simulink model "airspeed_controller"  (R2018b)
settings: Solver=FixedStepAuto  StartTime=0.0  StopTime=200  FixedStep=0.001  RelTol=1e-3
model workspace (MAT data in the model file):
  Cd = 0.18
  climb_max = 5
  g_common = 9.81
  mass_plane = 1.5
  nomThr = 0
  rou = 1.225
  sink_max = 1
  timeConstThrot = 8
libraries: simulink x2
settings Model: Creator=lee  LastModifiedBy=lee

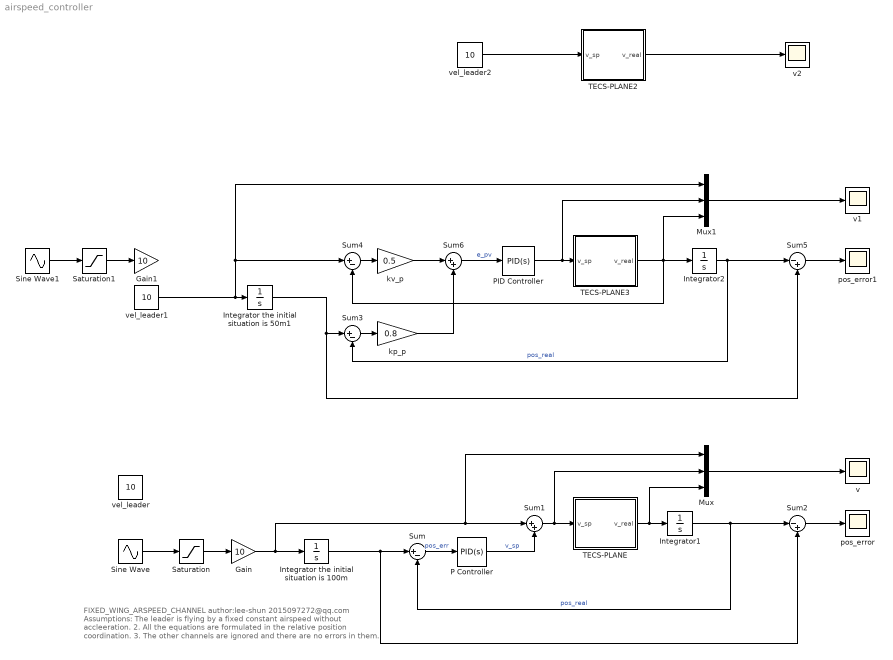
== system airspeed_controller ==
  note: FIXED_WING_ARSPEED_CHANNEL
      |
      | author:lee-shun 2015097272@qq.com
      |
      | Assumptions:
      |
      | The leader is flying by a fixed constant airspeed without accleeration.
      | 2. All the equations are formulated in the relative position coordination.
      | 3. The other channels are ignored and there are no errors in them.
  Gain : Gain  Gain=10
  Gain1 : Gain  Gain=10
  Integrator the initial situation is 100m : Integrator  InitialCondition=50  IgnoreLimit=on
  Integrator the initial situation is 50m1 : Integrator  InitialCondition=50  IgnoreLimit=on
  Integrator1 : Integrator
  Integrator2 : Integrator
  Mux : Mux  Inputs=3
  Mux1 : Mux  Inputs=3
  P Controller : simulink/Continuous/PID Controller  Controller=PID  Form=Parallel  TimeDomain=Continuous-time  SampleTime=-1  IntegratorMethod=Forward Euler  FilterMethod=Forward Euler  ControllerParametersSource=internal  P=0.02  I=0  D=0.0  UseFilter=on  N=100  TunerSelectOption=Transfer Function Based (PID Tuner App)  InitialConditionSource=internal  InitialConditionForIntegrator=0  InitialConditionForFilter=0  DifferentiatorICPrevScaledInput=0  ExternalReset=none  TrackingMode=off  Kt=1  LimitOutput=off  UpperSaturationLimit=inf  LowerSaturationLimit=-inf  LinearizeAsGain=on  AntiWindupMode=none  Kb=1  POutMin=[]  POutMax=[]  IOutMin=[]  IOutMax=[]  DOutMin=[]  DOutMax=[]  NOutMin=[]  NOutMax=[]  SumOutMin=[]  SumOutMax=[]  SaturationOutMin=[]  SaturationOutMax=[]  PParamMin=[]  PParamMax=[]  IParamMin=[]  IParamMax=[]  DParamMin=[]  DParamMax=[]  NParamMin=[]  NParamMax=[]  KbParamMin=[]  KbParamMax=[]  KtParamMin=[]  KtParamMax=[]  KbOutMin=[]  KbOutMax=[]  KtOutMin=[]  KtOutMax=[]  IntegratorOutMin=[]  IntegratorOutMax=[]  FilterOutMin=[]  FilterOutMax=[]  SumI1OutMin=[]  SumI1OutMax=[]  SumI2OutMin=[]  SumI2OutMax=[]  SumI3OutMin=[]  SumI3OutMax=[]  SumI4OutMin=[]  SumI4OutMax=[]  SumDOutMin=[]  SumDOutMax=[]  DifferentiatorOutMin=[]  DifferentiatorOutMax=[]  FilterDiffOutCoefMin=[]  FilterDiffOutCoefMax=[]  ReciprocalOutMin=[]  ReciprocalOutMax=[]  SumDenOutMin=[]  SumDenOutMax=[]  SumNumOutMin=[]  SumNumOutMax=[]  DivideOutMin=[]  DivideOutMax=[]  IntegratorContinuousStateAttributes=''  IntegratorStateMustResolveToSignalObject=off  IntegratorRTWStateStorageClass=Auto  FilterContinuousStateAttributes=''  FilterStateMustResolveToSignalObject=off  FilterRTWStateStorageClass=Auto  ParallelPVariant=InternalParameters  IdealPVariant=Disabled  IVariant=InternalParameters  DVariant=InternalParameters  IntegratorVariant=Continuous  SatVariant=Disabled  AWVariant=Passthrough  PCopyVariant=Disabled  TRVariant=Disabled  FdbkBlocksVariant=Forward  IdealPFdbkVariant=Disabled  SatFdbkVariant=Disabled  DerivativeFilterVariant=ContFilter  NVariant=InternalParameters  NCopyVariant=Disabled  FilterICVariant=InternalICsFilter  IntegratorICVariant=InternalICs  ExternalResetVariant=Disabled  TRSumVariant=Passthrough  SumFdbkVariant=Disabled  SumVariant=Sum_PID
  PID Controller : simulink/Continuous/PID Controller  Controller=PID  Form=Parallel  TimeDomain=Continuous-time  SampleTime=-1  IntegratorMethod=Forward Euler  FilterMethod=Forward Euler  ControllerParametersSource=internal  P=0.3  I=0.01  D=0  UseFilter=on  N=100  TunerSelectOption=Transfer Function Based (PID Tuner App)  InitialConditionSource=internal  InitialConditionForIntegrator=0  InitialConditionForFilter=0  DifferentiatorICPrevScaledInput=0  ExternalReset=none  TrackingMode=off  Kt=1  LimitOutput=off  UpperSaturationLimit=inf  LowerSaturationLimit=-inf  LinearizeAsGain=on  AntiWindupMode=none  Kb=1  POutMin=[]  POutMax=[]  IOutMin=[]  IOutMax=[]  DOutMin=[]  DOutMax=[]  NOutMin=[]  NOutMax=[]  SumOutMin=[]  SumOutMax=[]  SaturationOutMin=[]  SaturationOutMax=[]  PParamMin=[]  PParamMax=[]  IParamMin=[]  IParamMax=[]  DParamMin=[]  DParamMax=[]  NParamMin=[]  NParamMax=[]  KbParamMin=[]  KbParamMax=[]  KtParamMin=[]  KtParamMax=[]  KbOutMin=[]  KbOutMax=[]  KtOutMin=[]  KtOutMax=[]  IntegratorOutMin=[]  IntegratorOutMax=[]  FilterOutMin=[]  FilterOutMax=[]  SumI1OutMin=[]  SumI1OutMax=[]  SumI2OutMin=[]  SumI2OutMax=[]  SumI3OutMin=[]  SumI3OutMax=[]  SumI4OutMin=[]  SumI4OutMax=[]  SumDOutMin=[]  SumDOutMax=[]  DifferentiatorOutMin=[]  DifferentiatorOutMax=[]  FilterDiffOutCoefMin=[]  FilterDiffOutCoefMax=[]  ReciprocalOutMin=[]  ReciprocalOutMax=[]  SumDenOutMin=[]  SumDenOutMax=[]  SumNumOutMin=[]  SumNumOutMax=[]  DivideOutMin=[]  DivideOutMax=[]  IntegratorContinuousStateAttributes=''  IntegratorStateMustResolveToSignalObject=off  IntegratorRTWStateStorageClass=Auto  FilterContinuousStateAttributes=''  FilterStateMustResolveToSignalObject=off  FilterRTWStateStorageClass=Auto  ParallelPVariant=InternalParameters  IdealPVariant=Disabled  IVariant=InternalParameters  DVariant=InternalParameters  IntegratorVariant=Continuous  SatVariant=Disabled  AWVariant=Passthrough  PCopyVariant=Disabled  TRVariant=Disabled  FdbkBlocksVariant=Forward  IdealPFdbkVariant=Disabled  SatFdbkVariant=Disabled  DerivativeFilterVariant=ContFilter  NVariant=InternalParameters  NCopyVariant=Disabled  FilterICVariant=InternalICsFilter  IntegratorICVariant=InternalICs  ExternalResetVariant=Disabled  TRSumVariant=Passthrough  SumFdbkVariant=Disabled  SumVariant=Sum_PID
  Saturation : Saturate  UpperLimit=1  LowerLimit=0.2
  Saturation1 : Saturate  UpperLimit=1  LowerLimit=0.2
  Sine Wave : Sin  Frequency=0.1  SampleTime=0
  Sine Wave1 : Sin  Frequency=0.1  SampleTime=0
  Sum : Sum  Inputs=|+-
  Sum1 : Sum  Inputs=|++
  Sum2 : Sum  Inputs=|-+
  Sum3 : Sum  Inputs=|+-
  Sum4 : Sum  Inputs=|+-
  Sum5 : Sum  Inputs=|-+
  Sum6 : Sum  Inputs=|++
  TECS-PLANE : Subsystem
  TECS-PLANE2 : Subsystem
  TECS-PLANE3 : Subsystem
  kp_p : Gain  Gain=0.8
  kv_p : Gain  Gain=0.5
  pos_error : Scope
  pos_error1 : Scope
  v : Scope
  v1 : Scope
  v2 : Scope
  vel_leader : Constant  Value=10
  vel_leader1 : Constant  Value=10
  vel_leader2 : Constant  Value=10
  wires:
  Sum/1 -> P Controller/1  "pos_err"
  Integrator1/1 -> Sum/2, Sum2/1  "pos_real"
  Integrator the initial situation is 100m/1 -> Sum/1, Sum2/2
  TECS-PLANE/1(v_real) -> Mux/3, Integrator1/1
  P Controller/1 -> Sum1/2  "v_sp"
  Sum1/1 -> Mux/2, TECS-PLANE/1(v_sp)
  Sum2/1 -> pos_error/1
  Sine Wave/1 -> Saturation/1
  Saturation/1 -> Gain/1
  Gain/1 -> Mux/1, Sum1/1, Integrator the initial situation is 100m/1
  Mux/1 -> v/1
  Sum5/1 -> pos_error1/1
  Saturation1/1 -> Gain1/1
  Sine Wave1/1 -> Saturation1/1
  TECS-PLANE3/1(v_real) -> Integrator2/1, Mux1/3, Sum4/2
  Integrator2/1 -> Sum5/1, Sum3/2  "pos_real"
  Mux1/1 -> v1/1
  Integrator the initial situation is 50m1/1 -> Sum3/1, Sum5/2
  kv_p/1 -> Sum6/1
  Sum4/1 -> kv_p/1
  Sum3/1 -> kp_p/1
  kp_p/1 -> Sum6/2
  Sum6/1 -> PID Controller/1  "e_pv"
  PID Controller/1 -> TECS-PLANE3/1(v_sp), Mux1/2
  vel_leader1/1 -> Sum4/1, Mux1/1, Integrator the initial situation is 50m1/1
  vel_leader2/1 -> TECS-PLANE2/1(v_sp)
  TECS-PLANE2/1(v_real) -> v2/1

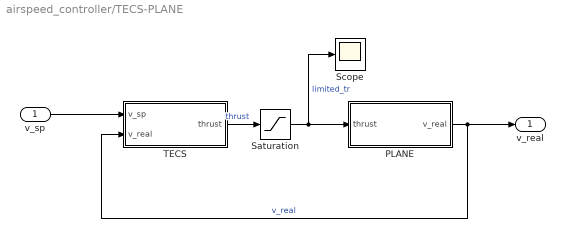
== system airspeed_controller/TECS-PLANE ==
  v_sp : Inport
  PLANE : Subsystem
  Saturation : Saturate  UpperLimit=1  LowerLimit=0  ZeroCross=off
  Scope : Scope
  "TECS " : Subsystem
  v_real : Outport  VectorParamsAs1DForOutWhenUnconnected=on
  wires:
  PLANE/1(v_real) -> v_real/1, "TECS "/2(v_real)  "v_real"
  Saturation/1 -> Scope/1, PLANE/1(thrust)  "limited_tr"
  "TECS "/1(thrust) -> Saturation/1  "thrust"
  v_sp/1 -> "TECS "/1(v_sp)

== system airspeed_controller/TECS-PLANE2 ==
  v_sp : Inport
  PLANE : Subsystem
  Saturation : Saturate  UpperLimit=1  LowerLimit=0  ZeroCross=off
  Scope : Scope
  "TECS " : Subsystem
  v_real : Outport  VectorParamsAs1DForOutWhenUnconnected=on
  wires:
  PLANE/1(v_real) -> v_real/1, "TECS "/2(v_real)  "v_real"
  Saturation/1 -> Scope/1, PLANE/1(thrust)  "limited_tr"
  "TECS "/1(thrust) -> Saturation/1  "thrust"
  v_sp/1 -> "TECS "/1(v_sp)

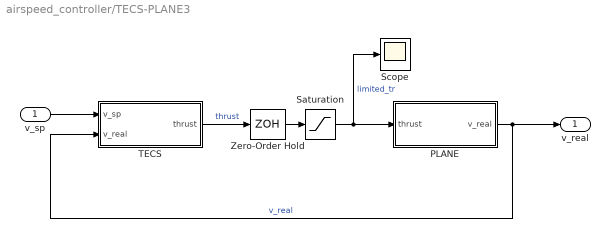
== system airspeed_controller/TECS-PLANE3 ==
  v_sp : Inport
  PLANE : Subsystem
  Saturation : Saturate  UpperLimit=1  LowerLimit=0  ZeroCross=off
  Scope : Scope
  "TECS " : Subsystem
  Zero-Order Hold : ZeroOrderHold  SampleTime=-1
  v_real : Outport  VectorParamsAs1DForOutWhenUnconnected=on
  wires:
  PLANE/1(v_real) -> v_real/1, "TECS "/2(v_real)  "v_real"
  Saturation/1 -> Scope/1, PLANE/1(thrust)  "limited_tr"
  "TECS "/1(thrust) -> Zero-Order Hold/1  "thrust"
  v_sp/1 -> "TECS "/1(v_sp)
  Zero-Order Hold/1 -> Saturation/1

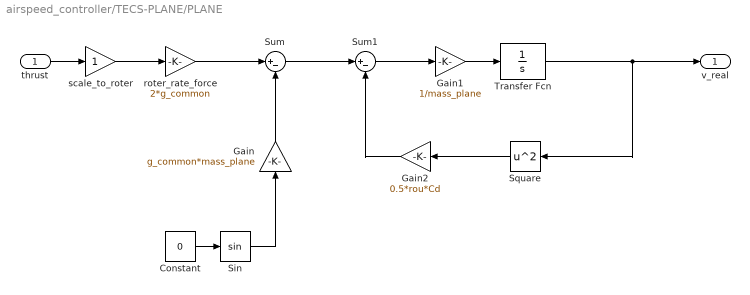
== system airspeed_controller/TECS-PLANE/PLANE ==
  thrust : Inport
  Constant : Constant  Value=0
  Gain : Gain  Gain=g_common*mass_plane
  Gain1 : Gain  Gain=1/mass_plane
  Gain2 : Gain  Gain=0.5*rou*Cd
  Sin : Trigonometry
  Square : Math  Operator=square  SaturateOnIntegerOverflow=on
  Sum : Sum  Inputs=|+-
  Sum1 : Sum  Inputs=|+-
  Transfer Fcn : TransferFcn  Denominator=[1 0]
  roter_rate_force : Gain  Gain=2*g_common
  scale_to_roter : Gain
  v_real : Outport  VectorParamsAs1DForOutWhenUnconnected=on
  wires:
  thrust/1 -> scale_to_roter/1
  scale_to_roter/1 -> roter_rate_force/1
  roter_rate_force/1 -> Sum/1
  Gain/1 -> Sum/2
  Constant/1 -> Sin/1
  Sin/1 -> Gain/1
  Sum/1 -> Sum1/1
  Sum1/1 -> Gain1/1
  Gain1/1 -> Transfer Fcn/1
  Transfer Fcn/1 -> Square/1, v_real/1
  Square/1 -> Gain2/1
  Gain2/1 -> Sum1/2

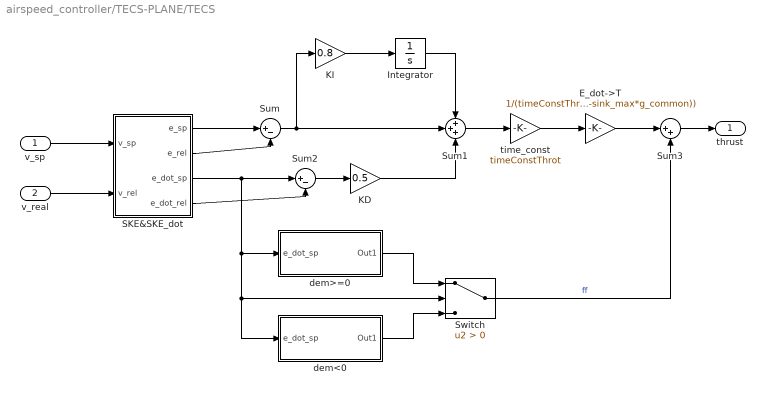
== system airspeed_controller/TECS-PLANE/TECS  ==
  v_sp : Inport
  v_real : Inport  Port=2
  E_dot->T : Gain  Gain=1/(timeConstThrot*(climb_max*g_common-sink_max*g_common))
  Integrator : Integrator
  KD : Gain  Gain=0.5
  KI : Gain  Gain=0.8
  SKE&SKE_dot : Subsystem
  Sum : Sum  Inputs=|+-
  Sum1 : Sum  Inputs=+++
  Sum2 : Sum  Inputs=|+-
  Sum3 : Sum  Inputs=|++
  Switch : Switch  Criteria=u2 > Threshold  ZeroCross=off
  dem<0 : Subsystem
  dem>=0 : Subsystem
  time_const : Gain  Gain=timeConstThrot
  thrust : Outport  VectorParamsAs1DForOutWhenUnconnected=on
  wires:
  Sum/1 -> Sum1/2, KI/1
  KI/1 -> Integrator/1
  Integrator/1 -> Sum1/1
  Sum1/1 -> time_const/1
  time_const/1 -> E_dot->T/1
  E_dot->T/1 -> Sum3/1
  v_sp/1 -> SKE&SKE_dot/1(v_sp)
  v_real/1 -> SKE&SKE_dot/2(v_rel)
  SKE&SKE_dot/1(e_sp) -> Sum/1
  SKE&SKE_dot/2(e_rel) -> Sum/2
  SKE&SKE_dot/3(e_dot_sp) -> dem<0/1(e_dot_sp), Switch/2, dem>=0/1(e_dot_sp), Sum2/1
  SKE&SKE_dot/4(e_dot_rel) -> Sum2/2
  Sum2/1 -> KD/1
  KD/1 -> Sum1/3
  Sum3/1 -> thrust/1
  Switch/1 -> Sum3/2  "ff"
  dem>=0/1(Out1) -> Switch/1
  dem<0/1(Out1) -> Switch/3

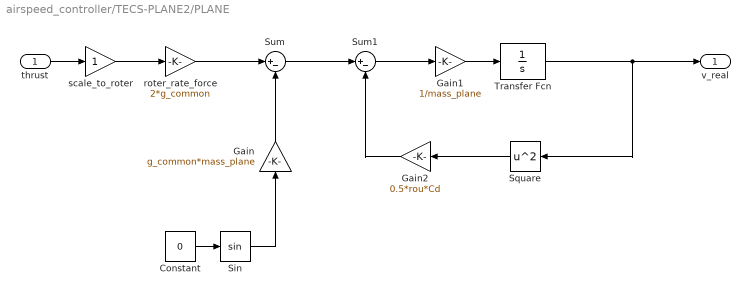
== system airspeed_controller/TECS-PLANE2/PLANE ==
  thrust : Inport
  Constant : Constant  Value=0
  Gain : Gain  Gain=g_common*mass_plane
  Gain1 : Gain  Gain=1/mass_plane
  Gain2 : Gain  Gain=0.5*rou*Cd
  Sin : Trigonometry
  Square : Math  Operator=square  SaturateOnIntegerOverflow=on
  Sum : Sum  Inputs=|+-
  Sum1 : Sum  Inputs=|+-
  Transfer Fcn : TransferFcn  Denominator=[1 0]
  roter_rate_force : Gain  Gain=2*g_common
  scale_to_roter : Gain
  v_real : Outport  VectorParamsAs1DForOutWhenUnconnected=on
  wires:
  thrust/1 -> scale_to_roter/1
  scale_to_roter/1 -> roter_rate_force/1
  roter_rate_force/1 -> Sum/1
  Gain/1 -> Sum/2
  Constant/1 -> Sin/1
  Sin/1 -> Gain/1
  Sum/1 -> Sum1/1
  Sum1/1 -> Gain1/1
  Gain1/1 -> Transfer Fcn/1
  Transfer Fcn/1 -> Square/1, v_real/1
  Square/1 -> Gain2/1
  Gain2/1 -> Sum1/2

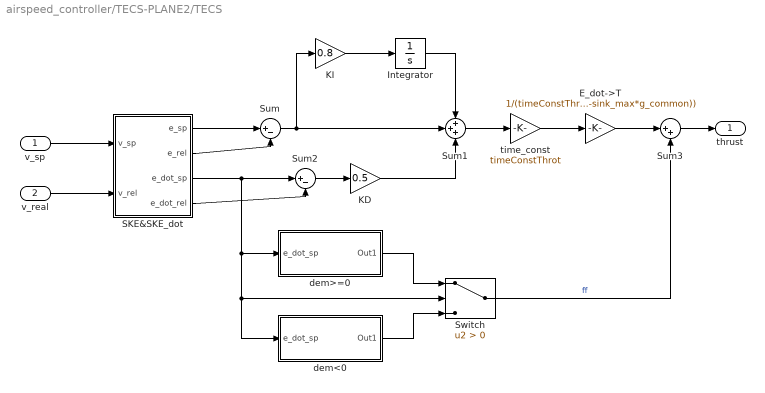
== system airspeed_controller/TECS-PLANE2/TECS  ==
  v_sp : Inport
  v_real : Inport  Port=2
  E_dot->T : Gain  Gain=1/(timeConstThrot*(climb_max*g_common-sink_max*g_common))
  Integrator : Integrator
  KD : Gain  Gain=0.5
  KI : Gain  Gain=0.8
  SKE&SKE_dot : Subsystem
  Sum : Sum  Inputs=|+-
  Sum1 : Sum  Inputs=+++
  Sum2 : Sum  Inputs=|+-
  Sum3 : Sum  Inputs=|++
  Switch : Switch  Criteria=u2 > Threshold  ZeroCross=off
  dem<0 : Subsystem
  dem>=0 : Subsystem
  time_const : Gain  Gain=timeConstThrot
  thrust : Outport  VectorParamsAs1DForOutWhenUnconnected=on
  wires:
  Sum/1 -> Sum1/2, KI/1
  KI/1 -> Integrator/1
  Integrator/1 -> Sum1/1
  Sum1/1 -> time_const/1
  time_const/1 -> E_dot->T/1
  E_dot->T/1 -> Sum3/1
  v_sp/1 -> SKE&SKE_dot/1(v_sp)
  v_real/1 -> SKE&SKE_dot/2(v_rel)
  SKE&SKE_dot/1(e_sp) -> Sum/1
  SKE&SKE_dot/2(e_rel) -> Sum/2
  SKE&SKE_dot/3(e_dot_sp) -> dem<0/1(e_dot_sp), Switch/2, dem>=0/1(e_dot_sp), Sum2/1
  SKE&SKE_dot/4(e_dot_rel) -> Sum2/2
  Sum2/1 -> KD/1
  KD/1 -> Sum1/3
  Sum3/1 -> thrust/1
  Switch/1 -> Sum3/2  "ff"
  dem>=0/1(Out1) -> Switch/1
  dem<0/1(Out1) -> Switch/3

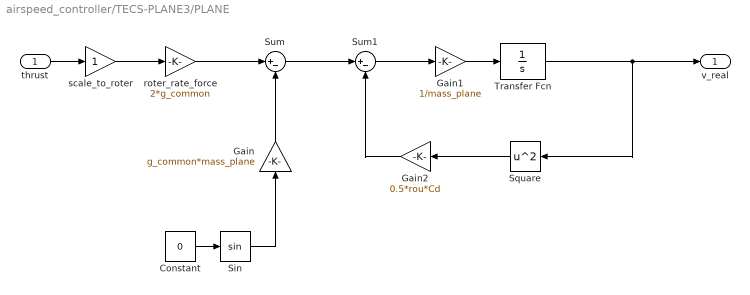
== system airspeed_controller/TECS-PLANE3/PLANE ==
  thrust : Inport
  Constant : Constant  Value=0
  Gain : Gain  Gain=g_common*mass_plane
  Gain1 : Gain  Gain=1/mass_plane
  Gain2 : Gain  Gain=0.5*rou*Cd
  Sin : Trigonometry
  Square : Math  Operator=square  SaturateOnIntegerOverflow=on
  Sum : Sum  Inputs=|+-
  Sum1 : Sum  Inputs=|+-
  Transfer Fcn : TransferFcn  Denominator=[1 0]
  roter_rate_force : Gain  Gain=2*g_common
  scale_to_roter : Gain
  v_real : Outport  VectorParamsAs1DForOutWhenUnconnected=on
  wires:
  thrust/1 -> scale_to_roter/1
  scale_to_roter/1 -> roter_rate_force/1
  roter_rate_force/1 -> Sum/1
  Gain/1 -> Sum/2
  Constant/1 -> Sin/1
  Sin/1 -> Gain/1
  Sum/1 -> Sum1/1
  Sum1/1 -> Gain1/1
  Gain1/1 -> Transfer Fcn/1
  Transfer Fcn/1 -> Square/1, v_real/1
  Square/1 -> Gain2/1
  Gain2/1 -> Sum1/2

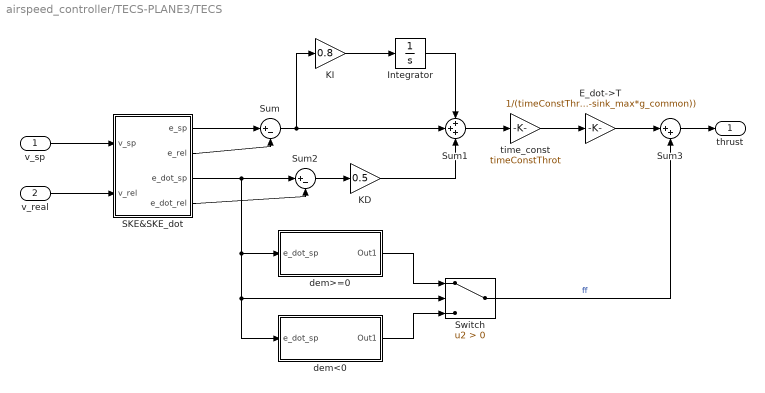
== system airspeed_controller/TECS-PLANE3/TECS  ==
  v_sp : Inport
  v_real : Inport  Port=2
  E_dot->T : Gain  Gain=1/(timeConstThrot*(climb_max*g_common-sink_max*g_common))
  Integrator : Integrator
  KD : Gain  Gain=0.5
  KI : Gain  Gain=0.8
  SKE&SKE_dot : Subsystem
  Sum : Sum  Inputs=|+-
  Sum1 : Sum  Inputs=+++
  Sum2 : Sum  Inputs=|+-
  Sum3 : Sum  Inputs=|++
  Switch : Switch  Criteria=u2 > Threshold  ZeroCross=off
  dem<0 : Subsystem
  dem>=0 : Subsystem
  time_const : Gain  Gain=timeConstThrot
  thrust : Outport  VectorParamsAs1DForOutWhenUnconnected=on
  wires:
  Sum/1 -> Sum1/2, KI/1
  KI/1 -> Integrator/1
  Integrator/1 -> Sum1/1
  Sum1/1 -> time_const/1
  time_const/1 -> E_dot->T/1
  E_dot->T/1 -> Sum3/1
  v_sp/1 -> SKE&SKE_dot/1(v_sp)
  v_real/1 -> SKE&SKE_dot/2(v_rel)
  SKE&SKE_dot/1(e_sp) -> Sum/1
  SKE&SKE_dot/2(e_rel) -> Sum/2
  SKE&SKE_dot/3(e_dot_sp) -> dem<0/1(e_dot_sp), Switch/2, dem>=0/1(e_dot_sp), Sum2/1
  SKE&SKE_dot/4(e_dot_rel) -> Sum2/2
  Sum2/1 -> KD/1
  KD/1 -> Sum1/3
  Sum3/1 -> thrust/1
  Switch/1 -> Sum3/2  "ff"
  dem>=0/1(Out1) -> Switch/1
  dem<0/1(Out1) -> Switch/3

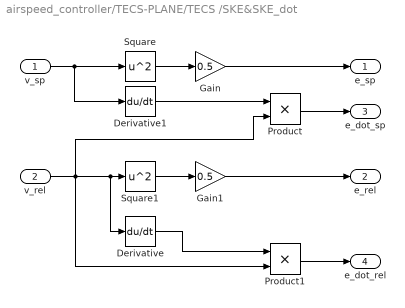
== system airspeed_controller/TECS-PLANE/TECS /SKE&SKE_dot ==
  v_sp : Inport
  v_rel : Inport  Port=2
  Derivative : Derivative
  Derivative1 : Derivative
  Gain : Gain  Gain=0.5
  Gain1 : Gain  Gain=0.5
  Product : Product
  Product1 : Product
  Square : Math  Operator=square  SaturateOnIntegerOverflow=on
  Square1 : Math  Operator=square  SaturateOnIntegerOverflow=on
  e_sp : Outport  VectorParamsAs1DForOutWhenUnconnected=on
  e_rel : Outport  Port=2  VectorParamsAs1DForOutWhenUnconnected=on
  e_dot_sp : Outport  Port=3  VectorParamsAs1DForOutWhenUnconnected=on
  e_dot_rel : Outport  Port=4  VectorParamsAs1DForOutWhenUnconnected=on
  wires:
  Square/1 -> Gain/1
  Square1/1 -> Gain1/1
  Gain/1 -> e_sp/1
  v_sp/1 -> Derivative1/1, Square/1
  Gain1/1 -> e_rel/1
  Product/1 -> e_dot_sp/1
  v_rel/1 -> Product1/2, Product/2, Derivative/1, Square1/1
  Product1/1 -> e_dot_rel/1
  Derivative1/1 -> Product/1
  Derivative/1 -> Product1/1

== system airspeed_controller/TECS-PLANE/TECS /dem<0 ==
  e_dot_sp : Inport
  Constant : Constant  Value=nomThr
  Gain : Gain  Gain=1/(sink_max*g_common)
  Gain1 : Gain  Gain=nomThr
  Sum : Sum  Inputs=|+-
  Out1 : Outport  VectorParamsAs1DForOutWhenUnconnected=on
  wires:
  Constant/1 -> Sum/1
  e_dot_sp/1 -> Gain/1
  Gain/1 -> Gain1/1
  Gain1/1 -> Sum/2
  Sum/1 -> Out1/1

== system airspeed_controller/TECS-PLANE/TECS /dem>=0 ==
  e_dot_sp : Inport
  Constant : Constant  Value=nomThr
  Gain : Gain  Gain=1/(climb_max*g_common)
  Gain1 : Gain  Gain=1-nomThr
  Sum : Sum  Inputs=|++
  Out1 : Outport  VectorParamsAs1DForOutWhenUnconnected=on
  wires:
  Constant/1 -> Sum/1
  e_dot_sp/1 -> Gain/1
  Gain/1 -> Gain1/1
  Gain1/1 -> Sum/2
  Sum/1 -> Out1/1

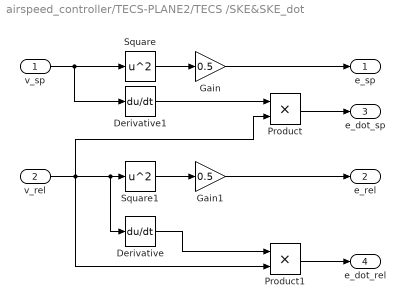
== system airspeed_controller/TECS-PLANE2/TECS /SKE&SKE_dot ==
  v_sp : Inport
  v_rel : Inport  Port=2
  Derivative : Derivative
  Derivative1 : Derivative
  Gain : Gain  Gain=0.5
  Gain1 : Gain  Gain=0.5
  Product : Product
  Product1 : Product
  Square : Math  Operator=square  SaturateOnIntegerOverflow=on
  Square1 : Math  Operator=square  SaturateOnIntegerOverflow=on
  e_sp : Outport  VectorParamsAs1DForOutWhenUnconnected=on
  e_rel : Outport  Port=2  VectorParamsAs1DForOutWhenUnconnected=on
  e_dot_sp : Outport  Port=3  VectorParamsAs1DForOutWhenUnconnected=on
  e_dot_rel : Outport  Port=4  VectorParamsAs1DForOutWhenUnconnected=on
  wires:
  Square/1 -> Gain/1
  Square1/1 -> Gain1/1
  Gain/1 -> e_sp/1
  v_sp/1 -> Derivative1/1, Square/1
  Gain1/1 -> e_rel/1
  Product/1 -> e_dot_sp/1
  v_rel/1 -> Product1/2, Product/2, Derivative/1, Square1/1
  Product1/1 -> e_dot_rel/1
  Derivative1/1 -> Product/1
  Derivative/1 -> Product1/1

== system airspeed_controller/TECS-PLANE2/TECS /dem<0 ==
  e_dot_sp : Inport
  Constant : Constant  Value=nomThr
  Gain : Gain  Gain=1/(sink_max*g_common)
  Gain1 : Gain  Gain=nomThr
  Sum : Sum  Inputs=|+-
  Out1 : Outport  VectorParamsAs1DForOutWhenUnconnected=on
  wires:
  Constant/1 -> Sum/1
  e_dot_sp/1 -> Gain/1
  Gain/1 -> Gain1/1
  Gain1/1 -> Sum/2
  Sum/1 -> Out1/1

== system airspeed_controller/TECS-PLANE2/TECS /dem>=0 ==
  e_dot_sp : Inport
  Constant : Constant  Value=nomThr
  Gain : Gain  Gain=1/(climb_max*g_common)
  Gain1 : Gain  Gain=1-nomThr
  Sum : Sum  Inputs=|++
  Out1 : Outport  VectorParamsAs1DForOutWhenUnconnected=on
  wires:
  Constant/1 -> Sum/1
  e_dot_sp/1 -> Gain/1
  Gain/1 -> Gain1/1
  Gain1/1 -> Sum/2
  Sum/1 -> Out1/1

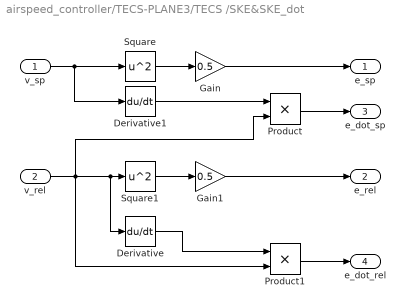
== system airspeed_controller/TECS-PLANE3/TECS /SKE&SKE_dot ==
  v_sp : Inport
  v_rel : Inport  Port=2
  Derivative : Derivative
  Derivative1 : Derivative
  Gain : Gain  Gain=0.5
  Gain1 : Gain  Gain=0.5
  Product : Product
  Product1 : Product
  Square : Math  Operator=square  SaturateOnIntegerOverflow=on
  Square1 : Math  Operator=square  SaturateOnIntegerOverflow=on
  e_sp : Outport  VectorParamsAs1DForOutWhenUnconnected=on
  e_rel : Outport  Port=2  VectorParamsAs1DForOutWhenUnconnected=on
  e_dot_sp : Outport  Port=3  VectorParamsAs1DForOutWhenUnconnected=on
  e_dot_rel : Outport  Port=4  VectorParamsAs1DForOutWhenUnconnected=on
  wires:
  Square/1 -> Gain/1
  Square1/1 -> Gain1/1
  Gain/1 -> e_sp/1
  v_sp/1 -> Derivative1/1, Square/1
  Gain1/1 -> e_rel/1
  Product/1 -> e_dot_sp/1
  v_rel/1 -> Product1/2, Product/2, Derivative/1, Square1/1
  Product1/1 -> e_dot_rel/1
  Derivative1/1 -> Product/1
  Derivative/1 -> Product1/1

== system airspeed_controller/TECS-PLANE3/TECS /dem<0 ==
  e_dot_sp : Inport
  Constant : Constant  Value=nomThr
  Gain : Gain  Gain=1/(sink_max*g_common)
  Gain1 : Gain  Gain=nomThr
  Sum : Sum  Inputs=|+-
  Out1 : Outport  VectorParamsAs1DForOutWhenUnconnected=on
  wires:
  Constant/1 -> Sum/1
  e_dot_sp/1 -> Gain/1
  Gain/1 -> Gain1/1
  Gain1/1 -> Sum/2
  Sum/1 -> Out1/1

== system airspeed_controller/TECS-PLANE3/TECS /dem>=0 ==
  e_dot_sp : Inport
  Constant : Constant  Value=nomThr
  Gain : Gain  Gain=1/(climb_max*g_common)
  Gain1 : Gain  Gain=1-nomThr
  Sum : Sum  Inputs=|++
  Out1 : Outport  VectorParamsAs1DForOutWhenUnconnected=on
  wires:
  Constant/1 -> Sum/1
  e_dot_sp/1 -> Gain/1
  Gain/1 -> Gain1/1
  Gain1/1 -> Sum/2
  Sum/1 -> Out1/1
